simulink model "EJ_01_j"  (R2018a)
settings: Solver=ode23t  StartTime=0.0  StopTime=5  FixedStep=0.01  MaxStep=0.05  RelTol=1e-3  EnableMultiTasking=on
PreLoadFcn:
  | mdl_puma560
values from neighbouring files (symbols this model uses):
  messi = RobotInit(pert)    [Ej_01.m]
  q0 = [0 -pi/2]    [Ej_01.m]
undefined symbols (not defined in the file or in its folder): slcoulomb
libraries: roblocks x5, simulink x1
settings Model: ExtModeTrigMode=oneshot  ExtModeArmWhenConnect=off  Creator=pic  LastModifiedBy=sebas
settings SolverCC: ZeroCrossControl=DisableAll
settings DataIOCC: SaveFormat=Array  SignalLoggingSaveFormat=ModelDataLogs  ReturnWorkspaceOutputs=on  TimeSaveName=t  OutputSaveName=y  ReturnWorkspaceOutputsName=ctorque
settings OptimizationCC: BlockReduction=off  BooleanDataType=off  ExpressionDepthLimit=2147483647  InitFltsAndDblsToZero=on  LifeSpan=inf
settings DebuggingCC: SaveWithParameterizedLinksMsg=none  UnderspecifiedInitializationDetection=Classic  MergeDetectMultiDrivingBlocksExec=none  SignalResolutionControl=TryResolveAllWithWarning  MultiTaskDSMMsg=warning  MultiTaskCondExecSysMsg=none  FcnCallInpInsideContextMsg=warning  AllowSymbolicDim=off  StateNameClashWarn=warning  SFUnexpectedBacktrackingDiag=warning  SFNoUnconditionalDefaultTransitionDiag=warning  SFExecutionAtInitializationDiag=none
settings HardwareCC: ProdBitPerPointer=32  ProdBitPerSizeT=32  ProdBitPerPtrDiffT=32  ProdLargestAtomicFloat=None  ProdIntDivRoundTo=Undefined  ProdEndianess=Unspecified  ProdWordSize=32  ProdHWDeviceType=32-bit Generic  TargetUnknown=on
settings ModelReferenceCC: PropagateSignalLabelsOutOfModel=off
settings CodeAppCC: StateflowObjectComments=on
settings GRTTargetCC: TargetLangStandard=C89/C90 (ANSI)  ModelReferenceCompliant=off  CompOptLevelCompliant=off  GeneratePreprocessorConditionals=Disable all  CombineOutputUpdateFcns=off  MatFileLogging=off  GRTInterface=on
settings ConfigComp: CovMetricSettings=dw  CovHtmlReporting=on  CovSaveCumulativeToWorkspaceVar=on  CovSaveSingleToWorkspaceVar=on  CovExternalEMLEnable=off

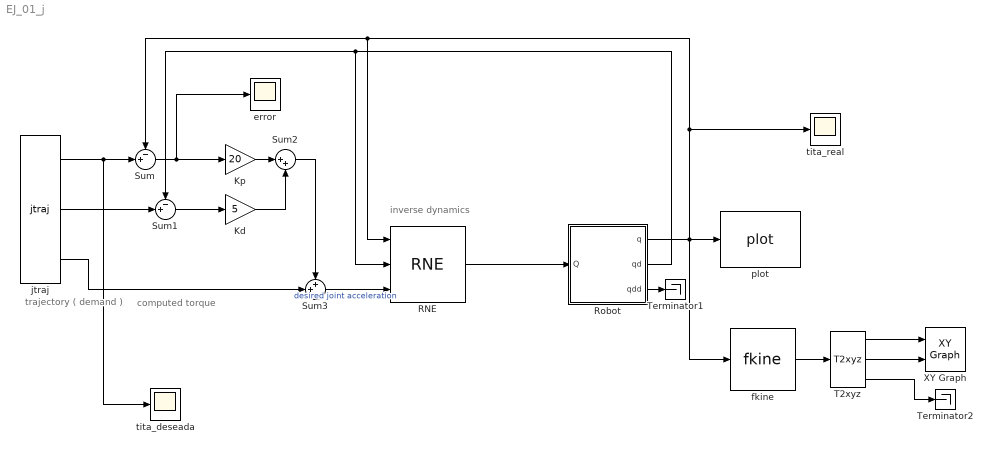
== system EJ_01_j ==
  note: inverse dynamics
  note: computed torque
  note: trajectory
      | ( demand )
  Kd : Gain  Gain=5  SaturateOnIntegerOverflow=on  OutDataTypeStr=Inherit: Same as input  ParamDataTypeStr=Inherit: Same as input
  Kp : Gain  Gain=20  SaturateOnIntegerOverflow=on  OutDataTypeStr=Inherit: Same as input  ParamDataTypeStr=Inherit: Same as input
  RNE : roblocks/Arm/RNE  robot=messi  grav=[0 0 9.81]
  Robot : Subsystem  AncestorBlock=roblocks/Arm/Robot  mask{robot=messi, q0=q0}
      mask prompts: robot "Robot object"; q0 "Initial state"
      mask help: Rigid-body dynamic model of robot.
      mask init:
      | if isa(robot, 'SerialLink')
      |     rname = robot.name;
      |     %fprintf('**robot name is %s\n', rname);
      | else
      |     rname = '';
      |     n = 0
      | end
      mask Help:
      | Simulates the forward (direct) rigid-body dynamics of the robot described
      | by the given robot object.  For given applied joint torque/force it computes
      | the instaneous joint coordinates, velocities and acclerations.
      | 
      | 
      | <b>Parameters::</b>
      | 
      | robot (SerialLink) a dynamic model of an N-link serial link manipulator
      | q0 (1xN)  Initial joint coordinates
      | 
      | <b>Inputs::</b>
      | 
      | Q (1xN) the generalized joint force (torque or force) required to achieve
      | the motion state (q, qd, qdd).
      | 
      | <b>Outputs::</b>
      | 
      | q (1xN) joint coordinates
      | qd (1xN) joint coordinate velocity
      | qdd (1xN) joint coordinate acceleration
      | 
      | 
      | <b>Notes::</b>
      | 
      | - Required to simulate robot rigid body motion.
      | - Implemented using the recursive Newton-Euler scheme (RNE).
      | - A wrapper for the Toolbox method accel() which in turn depends on the
      |   method rne().
      mask Display:
      | port_label('input', 1, 'Q')
      | port_label('output', 1, 'q')
      | port_label('output', 2, 'qd')
      | port_label('output', 3, 'qdd')
      | text(0.1, 0.9,  rname, 'horizontalAlignment', 'left')
  Sum : Sum  Inputs=-+|  SaturateOnIntegerOverflow=on  InputSameDT=on  OutDataTypeStr=Inherit: Same as first input
  Sum1 : Sum  Inputs=-+|  SaturateOnIntegerOverflow=on  InputSameDT=on  OutDataTypeStr=Inherit: Same as first input
  Sum2 : Sum  Inputs=|++  SaturateOnIntegerOverflow=on  InputSameDT=on  OutDataTypeStr=Inherit: Same as first input
  Sum3 : Sum  Inputs=++|  SaturateOnIntegerOverflow=on  InputSameDT=on  OutDataTypeStr=Inherit: Same as first input
  T2xyz : roblocks/Toolbox/T2xyz
  Terminator1 : Terminator
  Terminator2 : Terminator
  XY Graph : simulink/Sinks/XY Graph  xmin=0  xmax=1.5  ymin=-1.5  ymax=1.5  st=-1
  error : Scope
  fkine : roblocks/Arm/fkine  robot=messi
  jtraj : roblocks/Toolbox/jtraj  q0=q1  qf=q2  tmax=5  ts=-1
  plot : roblocks/Arm/plot  robot=messi  fps=10  holdplot=on
  tita_deseada : Scope
  tita_real : Scope
  wires:
  Sum/1 -> error/1, Kp/1
  Kp/1 -> Sum2/1
  Robot/1(q) -> fkine/1, RNE/1, Sum/1, tita_real/1, plot/1
  jtraj/1 -> tita_deseada/1, Sum/2
  jtraj/2 -> Sum1/2
  Sum1/1 -> Kd/1
  Kd/1 -> Sum2/2
  Robot/3(qdd) -> Terminator1/1
  Sum3/1 -> RNE/3  "desired joint acceleration"
  RNE/1 -> Robot/1(Q)
  Robot/2(qd) -> RNE/2, Sum1/1
  jtraj/3 -> Sum3/2
  Sum2/1 -> Sum3/1
  fkine/1 -> T2xyz/1
  T2xyz/1 -> XY Graph/1
  T2xyz/2 -> XY Graph/2
  T2xyz/3 -> Terminator2/1

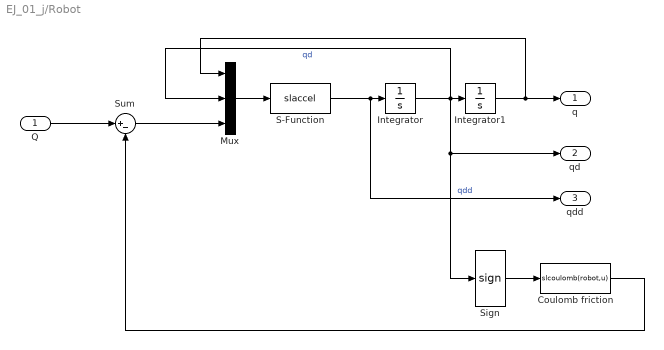
== system EJ_01_j/Robot ==
  Q : Inport
  Coulomb friction : MATLABFcn  MATLABFcn=slcoulomb(robot,u)  OutputDimensions=[robot.n 1]  Output1D=off
  Integrator : Integrator
  Integrator1 : Integrator  InitialCondition=q0
  Mux : Mux  Inputs=3
  S-Function : S-Function  FunctionName=slaccel  Parameters=robot  SFunctionDeploymentMode=off  EnableBusSupport=off
  Sign : Signum
  Sum : Sum  Inputs=|+-
  q : Outport
  qd : Outport  Port=2
  qdd : Outport  Port=3
  wires:
  S-Function/1 -> qdd/1, Integrator/1  "qdd"
  Mux/1 -> S-Function/1
  Integrator/1 -> Sign/1, qd/1, Integrator1/1, Mux/2  "qd"
  Integrator1/1 -> q/1, Mux/1
  Q/1 -> Sum/1
  Sum/1 -> Mux/3
  Coulomb friction/1 -> Sum/2
  Sign/1 -> Coulomb friction/1
